simulink model "gm_test_prediction_without_delays"  (R2022a)
settings: Solver=FixedStepDiscrete  StartTime=0.0  StopTime=10.0  RelTol=1e-3
undefined symbols (not defined in the file or in its folder): f_c, L_d, L_q, L_x, L_y, p, psi_pm, R_ph
libraries: hdlmdlgenlib x2
(part 3 of 9)

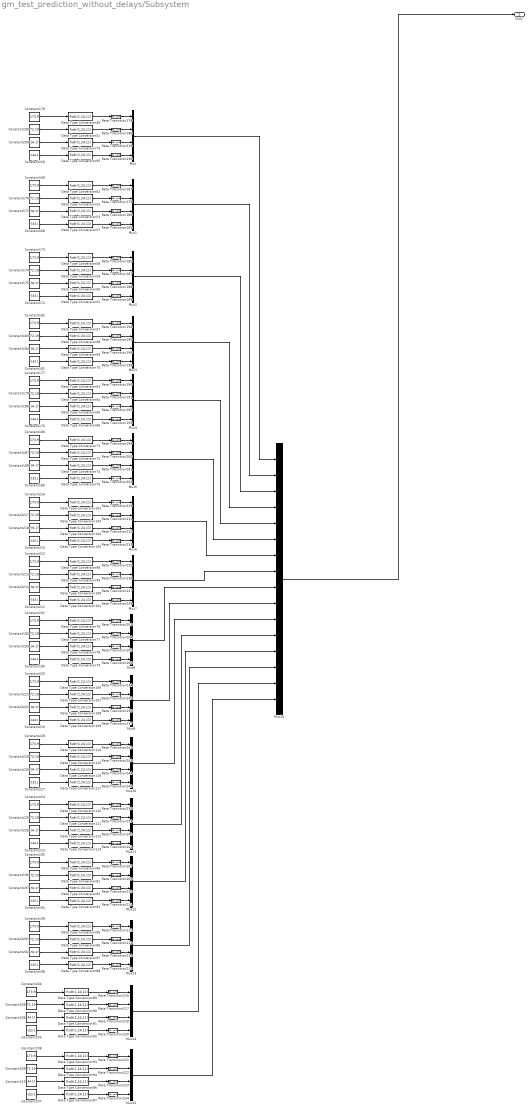
== system gm_test_prediction_without_delays/Subsystem ==
  Constant{156,168,172,176,181,185,190,194,198,203,207,211,215,219,223,227} (16 alike) : Constant  Value=-163.1
  Constant{169,173,177..178,182,186,191,195,199,204,208,212,216,220,224,228} (16 alike) : Constant  Value=173.9
  Constant{170,174,179,183,187,189,192,196,201,205,209,213,217,221,225,229} (16 alike) : Constant  Value=72.19
  Constant{171,175,180,184,188,193,197,200,202,206,210,214,218,222,226,230} (16 alike) : Constant  Value=-94.17
  Data Type Conversion{46,51..53,57..83,85..117} (64 alike) : DataTypeConversion  OutDataTypeStr=fixdt(1,24,11)  SaturateOnIntegerOverflow=off  RndMeth=Floor
  Mux{,1..15} (16 alike) : Mux
  Mux16 : Mux  Inputs=16
  Rate Transition{167,178..180,184..196,198..207,209..245} (64 alike) : RateTransition  OutPortSampleTime=Rt
  Out1 : Outport
  wires:
  Mux16/1 -> Out1/1
  Data Type Conversion65/1 -> Rate Transition192/1
  Data Type Conversion100/1 -> Rate Transition227/1
  Mux13/1 -> Mux16/14
  Constant204/1 -> Data Type Conversion89/1
  Rate Transition212/1 -> Mux13/1
  Constant220/1 -> Data Type Conversion106/1
  Constant202/1 -> Data Type Conversion87/1
  Constant218/1 -> Data Type Conversion104/1
  Rate Transition238/1 -> Mux11/1
  Constant224/1 -> Data Type Conversion110/1
  Rate Transition223/1 -> Mux15/3
  Constant177/1 -> Data Type Conversion63/1
  Constant183/1 -> Data Type Conversion68/1
  Data Type Conversion97/1 -> Rate Transition224/1
  Constant176/1 -> Data Type Conversion66/1
  Data Type Conversion74/1 -> Rate Transition201/1
  Data Type Conversion105/1 -> Rate Transition233/1
  Constant196/1 -> Data Type Conversion81/1
  Constant198/1 -> Data Type Conversion88/1
  Data Type Conversion115/1 -> Rate Transition243/1
  Constant225/1 -> Data Type Conversion111/1
  Constant222/1 -> Data Type Conversion108/1
  Data Type Conversion104/1 -> Rate Transition232/1
  Constant229/1 -> Data Type Conversion115/1
  Constant217/1 -> Data Type Conversion103/1
  Data Type Conversion72/1 -> Rate Transition200/1
  Data Type Conversion117/1 -> Rate Transition245/1
  Constant223/1 -> Data Type Conversion113/1
  Constant174/1 -> Data Type Conversion59/1
  Data Type Conversion110/1 -> Rate Transition238/1
  Data Type Conversion89/1 -> Rate Transition216/1
  Constant207/1 -> Data Type Conversion97/1
  Rate Transition185/1 -> Mux2/1
  Rate Transition196/1 -> Mux3/3
  Rate Transition230/1 -> Mux/4
  Data Type Conversion91/1 -> Rate Transition218/1
  Rate Transition167/1 -> Mux1/1
  Data Type Conversion85/1 -> Rate Transition212/1
  Rate Transition219/1 -> Mux/3
  Data Type Conversion102/1 -> Rate Transition229/1
  Constant156/1 -> Data Type Conversion95/1
  Constant228/1 -> Data Type Conversion114/1
  Rate Transition198/1 -> Mux3/4
  Rate Transition200/1 -> Mux5/2
  Data Type Conversion111/1 -> Rate Transition239/1
  Rate Transition192/1 -> Mux4/3
  Rate Transition190/1 -> Mux4/1
  Constant210/1 -> Data Type Conversion96/1
  Constant170/1 -> Data Type Conversion52/1
  Rate Transition195/1 -> Mux3/2
  Constant209/1 -> Data Type Conversion94/1
  Data Type Conversion93/1 -> Rate Transition221/1
  Data Type Conversion67/1 -> Rate Transition194/1
  Data Type Conversion73/1 -> Rate Transition219/1
  Constant184/1 -> Data Type Conversion69/1
  Rate Transition184/1 -> Mux1/4
  Data Type Conversion70/1 -> Rate Transition198/1
  Constant182/1 -> Data Type Conversion67/1
  Data Type Conversion75/1 -> Rate Transition202/1
  Constant189/1 -> Data Type Conversion51/1
  Constant206/1 -> Data Type Conversion91/1
  Constant192/1 -> Data Type Conversion77/1
  Data Type Conversion83/1 -> Rate Transition211/1
  Data Type Conversion59/1 -> Rate Transition187/1
  Mux14/1 -> Mux16/15
  Rate Transition241/1 -> Mux11/4
  Data Type Conversion107/1 -> Rate Transition235/1
  Rate Transition213/1 -> Mux13/2
  Constant172/1 -> Data Type Conversion61/1
  Constant221/1 -> Data Type Conversion107/1
  Data Type Conversion57/1 -> Rate Transition184/1
  Data Type Conversion61/1 -> Rate Transition189/1
  Constant197/1 -> Data Type Conversion82/1
  Rate Transition231/1 -> Mux6/2
  Constant173/1 -> Data Type Conversion58/1
  Constant190/1 -> Data Type Conversion79/1
  Constant230/1 -> Data Type Conversion116/1
  Constant193/1 -> Data Type Conversion78/1
  Rate Transition189/1 -> Mux2/4
  Rate Transition240/1 -> Mux11/3
  Rate Transition226/1 -> Mux7/2
  Data Type Conversion112/1 -> Rate Transition240/1
  Rate Transition239/1 -> Mux11/2
  Constant211/1 -> Data Type Conversion101/1
  Constant213/1 -> Data Type Conversion99/1
  Mux15/1 -> Mux16/16
  Data Type Conversion109/1 -> Rate Transition237/1
  Data Type Conversion46/1 -> Rate Transition178/1
  Data Type Conversion63/1 -> Rate Transition190/1
  Constant191/1 -> Data Type Conversion76/1
  Data Type Conversion80/1 -> Rate Transition207/1
  Constant168/1 -> Data Type Conversion57/1
  Constant195/1 -> Data Type Conversion80/1
  Constant194/1 -> Data Type Conversion83/1
  Data Type Conversion101/1 -> Rate Transition228/1
  Data Type Conversion77/1 -> Rate Transition204/1
  Data Type Conversion88/1 -> Rate Transition215/1
  Data Type Conversion96/1 -> Rate Transition223/1
  Rate Transition179/1 -> Mux1/2
  Data Type Conversion62/1 -> Rate Transition167/1
  Rate Transition234/1 -> Mux9/1
  Constant175/1 -> Data Type Conversion60/1
  Rate Transition225/1 -> Mux7/1
  Rate Transition218/1 -> Mux14/3
  Rate Transition220/1 -> Mux14/4
  Mux7/1 -> Mux16/8
  Rate Transition206/1 -> Mux8/4
  Data Type Conversion66/1 -> Rate Transition193/1
  Constant186/1 -> Data Type Conversion71/1
  Data Type Conversion98/1 -> Rate Transition225/1
  Rate Transition178/1 -> Mux/1
  Data Type Conversion81/1 -> Rate Transition209/1
  Data Type Conversion108/1 -> Rate Transition236/1
  Rate Transition237/1 -> Mux9/4
  Mux10/1 -> Mux16/11
  Constant205/1 -> Data Type Conversion90/1
  Mux4/1 -> Mux16/5
  Rate Transition245/1 -> Mux10/4
  Data Type Conversion52/1 -> Rate Transition179/1
  Rate Transition243/1 -> Mux10/2
  Constant208/1 -> Data Type Conversion93/1
  Constant185/1 -> Data Type Conversion75/1
  Constant216/1 -> Data Type Conversion102/1
  Data Type Conversion76/1 -> Rate Transition203/1
  Constant199/1 -> Data Type Conversion85/1
  Rate Transition209/1 -> Mux12/2
  Constant214/1 -> Data Type Conversion100/1
  Constant226/1 -> Data Type Conversion112/1
  Rate Transition228/1 -> Mux7/4
  Data Type Conversion69/1 -> Rate Transition196/1
  Constant201/1 -> Data Type Conversion86/1
  Constant171/1 -> Data Type Conversion53/1
  Rate Transition227/1 -> Mux7/3
  Rate Transition210/1 -> Mux12/3
  Rate Transition235/1 -> Mux9/2
  Rate Transition211/1 -> Mux12/4
  Mux8/1 -> Mux16/9
  Data Type Conversion79/1 -> Rate Transition206/1
  Mux1/1 -> Mux16/2
  Constant215/1 -> Data Type Conversion105/1
  Mux/1 -> Mux16/1
  Constant227/1 -> Data Type Conversion117/1
  Data Type Conversion68/1 -> Rate Transition195/1
  Constant178/1 -> Data Type Conversion46/1
  Mux6/1 -> Mux16/7
  Data Type Conversion53/1 -> Rate Transition180/1
  Data Type Conversion114/1 -> Rate Transition242/1
  Rate Transition232/1 -> Mux6/3
  Rate Transition224/1 -> Mux15/4
  Rate Transition186/1 -> Mux/2
  Rate Transition242/1 -> Mux10/1
  Rate Transition193/1 -> Mux4/4
  Rate Transition204/1 -> Mux8/2
  Constant212/1 -> Data Type Conversion98/1
  Constant181/1 -> Data Type Conversion70/1
  Rate Transition202/1 -> Mux5/4
  Rate Transition233/1 -> Mux6/4
  Data Type Conversion82/1 -> Rate Transition210/1
  Rate Transition188/1 -> Mux2/3
  Rate Transition216/1 -> Mux14/1
  Rate Transition244/1 -> Mux10/3
  Constant180/1 -> Data Type Conversion65/1
  Mux5/1 -> Mux16/6
  Constant219/1 -> Data Type Conversion109/1
  Data Type Conversion116/1 -> Rate Transition244/1
  Rate Transition203/1 -> Mux8/1
  Rate Transition215/1 -> Mux13/4
  Rate Transition205/1 -> Mux8/3
  Rate Transition194/1 -> Mux3/1
  Rate Transition229/1 -> Mux6/1
  Constant188/1 -> Data Type Conversion74/1
  Mux11/1 -> Mux16/12
  Mux9/1 -> Mux16/10
  Rate Transition221/1 -> Mux15/1
  Constant200/1 -> Data Type Conversion73/1
  Constant179/1 -> Data Type Conversion64/1
  Data Type Conversion94/1 -> Rate Transition222/1
  Mux2/1 -> Mux16/3
  Constant203/1 -> Data Type Conversion92/1
  Rate Transition217/1 -> Mux14/2
  Rate Transition191/1 -> Mux4/2
  Data Type Conversion99/1 -> Rate Transition226/1
  Constant187/1 -> Data Type Conversion72/1
  Data Type Conversion51/1 -> Rate Transition186/1
  Data Type Conversion71/1 -> Rate Transition199/1
  Data Type Conversion106/1 -> Rate Transition234/1
  Data Type Conversion86/1 -> Rate Transition213/1
  Data Type Conversion78/1 -> Rate Transition205/1
  Rate Transition199/1 -> Mux5/1
  Mux3/1 -> Mux16/4
  Rate Transition180/1 -> Mux1/3
  Rate Transition236/1 -> Mux9/3
  Rate Transition214/1 -> Mux13/3
  Data Type Conversion92/1 -> Rate Transition220/1
  Data Type Conversion64/1 -> Rate Transition191/1
  Data Type Conversion90/1 -> Rate Transition217/1
  Data Type Conversion87/1 -> Rate Transition214/1
  Data Type Conversion58/1 -> Rate Transition185/1
  Rate Transition187/1 -> Mux2/2
  Data Type Conversion60/1 -> Rate Transition188/1
  Rate Transition207/1 -> Mux12/1
  Data Type Conversion113/1 -> Rate Transition241/1
  Mux12/1 -> Mux16/13
  Data Type Conversion103/1 -> Rate Transition231/1
  Rate Transition201/1 -> Mux5/3
  Rate Transition222/1 -> Mux15/2
  Data Type Conversion95/1 -> Rate Transition230/1
  Constant169/1 -> Data Type Conversion62/1

== system gm_test_prediction_without_delays/Prediction_and_cost_function1/Compare To Constant ==
  u : Inport  OutDataTypeStr=fixdt(1,32,0,'DataTypeOverride', 'Off')  SampleTime=1e-08
  Compare : RelationalOperator  Operator=<=  OutDataTypeStr=boolean
  Constant : Constant  DisableCoverage=on  Value=const  OutDataTypeStr=Inherit: Inherit via back propagation  SampleTime=-1
  y : Outport  SampleTime=1e-08
  wires:
  Compare/1 -> y/1
  Constant/1 -> Compare/2
  u/1 -> Compare/1

== system gm_test_prediction_without_delays/Prediction_and_cost_function1/Data Type Conversion1 ==
  In1 : Inport
  Data Type Conversion1 : DataTypeConversion  OutDataTypeStr=single  RndMeth=Nearest  SampleTime=1e-08  SaturateOnIntegerOverflow=off
  Data Type Conversion1_pd1 : Delay  DelayLength=6
  Out1 : Outport
  wires:
  In1/1 -> Data Type Conversion1/1
  Data Type Conversion1/1 -> Data Type Conversion1_pd1/1
  Data Type Conversion1_pd1/1 -> Out1/1

== system gm_test_prediction_without_delays/Prediction_and_cost_function1/Data Type Conversion10 ==
  In1 : Inport
  Data Type Conversion10 : DataTypeConversion  OutDataTypeStr=single  RndMeth=Nearest  SampleTime=1e-08  SaturateOnIntegerOverflow=off
  Data Type Conversion10_pd1 : Delay  DelayLength=6
  Out1 : Outport
  wires:
  In1/1 -> Data Type Conversion10/1
  Data Type Conversion10/1 -> Data Type Conversion10_pd1/1
  Data Type Conversion10_pd1/1 -> Out1/1

== system gm_test_prediction_without_delays/Prediction_and_cost_function1/Data Type Conversion18 ==
  In1 : Inport
  Data Type Conversion18 : DataTypeConversion  OutDataTypeStr=fixdt(1, 18, 11)  RndMeth=Nearest  SampleTime=1e-08  SaturateOnIntegerOverflow=off
  Data Type Conversion18_pd1 : Delay  DelayLength=6
  Out1 : Outport
  wires:
  In1/1 -> Data Type Conversion18/1
  Data Type Conversion18/1 -> Data Type Conversion18_pd1/1
  Data Type Conversion18_pd1/1 -> Out1/1

== system gm_test_prediction_without_delays/Prediction_and_cost_function1/Data Type Conversion4 ==
  In1 : Inport
  Data Type Conversion4 : DataTypeConversion  OutDataTypeStr=single  RndMeth=Nearest  SampleTime=1e-08  SaturateOnIntegerOverflow=off
  Data Type Conversion4_pd1 : Delay  DelayLength=6
  Out1 : Outport
  wires:
  In1/1 -> Data Type Conversion4/1
  Data Type Conversion4/1 -> Data Type Conversion4_pd1/1
  Data Type Conversion4_pd1/1 -> Out1/1

== system gm_test_prediction_without_delays/Prediction_and_cost_function1/Data Type Conversion7 ==
  In1 : Inport
  Data Type Conversion7 : DataTypeConversion  OutDataTypeStr=single  RndMeth=Nearest  SampleTime=1e-08  SaturateOnIntegerOverflow=off
  Data Type Conversion7_pd1 : Delay  DelayLength=6
  Out1 : Outport
  wires:
  In1/1 -> Data Type Conversion7/1
  Data Type Conversion7/1 -> Data Type Conversion7_pd1/1
  Data Type Conversion7_pd1/1 -> Out1/1

== system gm_test_prediction_without_delays/Prediction_and_cost_function1/Data Type Conversion8 ==
  In1 : Inport
  Data Type Conversion8 : DataTypeConversion  OutDataTypeStr=single  RndMeth=Nearest  SampleTime=1e-08  SaturateOnIntegerOverflow=off
  Data Type Conversion8_pd1 : Delay  DelayLength=6
  Out1 : Outport
  wires:
  In1/1 -> Data Type Conversion8/1
  Data Type Conversion8/1 -> Data Type Conversion8_pd1/1
  Data Type Conversion8_pd1/1 -> Out1/1

== system gm_test_prediction_without_delays/Prediction_and_cost_function1/Data Type Conversion9 ==
  In1 : Inport
  Data Type Conversion9 : DataTypeConversion  OutDataTypeStr=single  RndMeth=Nearest  SampleTime=1e-08  SaturateOnIntegerOverflow=off
  Data Type Conversion9_pd1 : Delay  DelayLength=6
  Out1 : Outport
  wires:
  In1/1 -> Data Type Conversion9/1
  Data Type Conversion9/1 -> Data Type Conversion9_pd1/1
  Data Type Conversion9_pd1/1 -> Out1/1

== system gm_test_prediction_without_delays/Prediction_and_cost_function1/Detect Rise Positive ==
  note: Edge
  note: U(k)
  U : Inport  OutDataTypeStr=boolean  SampleTime=1e-08
  Delay Input1 : UnitDelay  Description=Store in Global RAM  DisableCoverage=on  InitialCondition=vinit  SampleTime=-1  HasFrameUpgradeWarning=on
  FixPt Relational Operator : RelationalOperator  Operator=>  OutDataTypeStr=boolean  ZeroCross=off  InputSameDT=off
  Positive : Subsystem  mask(Compare To Zero){relop=>, OutDataTypeStr=boolean, ZeroCross=off}
      mask prompts: relop "Simulink:masks:Operator_MP"; OutDataTypeStr "Simulink:masks:OutputDataType_MP"; ZeroCross "Simulink:masks:EnableZerocrossingDetection_MP"
      mask help: Simulink:masks:CompareToZero_MD
      mask init:
      | OutDataTypeStr = 'boolean';
      | ZeroCross = 'off';
      | blkName = 'test_prediction_without_delays/Prediction_and_cost_function1/Detect Rise\nPositive/Positive';
      | relop = '>';
      | setValue = 'boolean';
      mask TypeOptions relop: == | ~= | < | <= | >= | >
      mask TypeOptions OutDataTypeStr: Simulink:masks:uint8 | Simulink:masks:boolean
      mask Callback ZeroCross: sl('zeroCrossEnable', gcbh);
      mask Display: disp([relop,' 0'])
  Y : Outport  SampleTime=1e-08
  wires:
  Delay Input1/1 -> FixPt Relational Operator/2
  FixPt Relational Operator/1 -> Y/1
  Positive/1(y) -> FixPt Relational Operator/1, Delay Input1/1
  U/1 -> Positive/1(u)

== system gm_test_prediction_without_delays/Prediction_and_cost_function1/Detect Rise Positive1 ==
  note: Edge
  note: U(k)
  U : Inport  OutDataTypeStr=boolean  SampleTime=1e-08
  Delay Input1 : UnitDelay  Description=Store in Global RAM  DisableCoverage=on  InitialCondition=vinit  SampleTime=-1  HasFrameUpgradeWarning=on
  FixPt Relational Operator : RelationalOperator  Operator=>  OutDataTypeStr=boolean  ZeroCross=off  InputSameDT=off
  Positive : Subsystem  mask(Compare To Zero){relop=>, OutDataTypeStr=boolean, ZeroCross=off}
      mask prompts: relop "Simulink:masks:Operator_MP"; OutDataTypeStr "Simulink:masks:OutputDataType_MP"; ZeroCross "Simulink:masks:EnableZerocrossingDetection_MP"
      mask help: Simulink:masks:CompareToZero_MD
      mask init:
      | OutDataTypeStr = 'boolean';
      | ZeroCross = 'off';
      | blkName = 'test_prediction_without_delays/Prediction_and_cost_function1/Detect Rise\nPositive1/Positive';
      | relop = '>';
      | setValue = 'boolean';
      mask TypeOptions relop: == | ~= | < | <= | >= | >
      mask TypeOptions OutDataTypeStr: Simulink:masks:uint8 | Simulink:masks:boolean
      mask Callback ZeroCross: sl('zeroCrossEnable', gcbh);
      mask Display: disp([relop,' 0'])
  Y : Outport  SampleTime=1e-08
  wires:
  Delay Input1/1 -> FixPt Relational Operator/2
  FixPt Relational Operator/1 -> Y/1
  Positive/1(y) -> FixPt Relational Operator/1, Delay Input1/1
  U/1 -> Positive/1(u)

== system gm_test_prediction_without_delays/Prediction_and_cost_function1/Detect Rise Positive2 ==
  note: Edge
  note: U(k)
  U : Inport  OutDataTypeStr=boolean  SampleTime=1e-08
  Delay Input1 : UnitDelay  Description=Store in Global RAM  DisableCoverage=on  InitialCondition=vinit  SampleTime=-1  HasFrameUpgradeWarning=on
  FixPt Relational Operator : RelationalOperator  Operator=>  OutDataTypeStr=boolean  ZeroCross=off  InputSameDT=off
  Positive : Subsystem  mask(Compare To Zero){relop=>, OutDataTypeStr=boolean, ZeroCross=off}
      mask prompts: relop "Simulink:masks:Operator_MP"; OutDataTypeStr "Simulink:masks:OutputDataType_MP"; ZeroCross "Simulink:masks:EnableZerocrossingDetection_MP"
      mask help: Simulink:masks:CompareToZero_MD
      mask init:
      | OutDataTypeStr = 'boolean';
      | ZeroCross = 'off';
      | blkName = 'test_prediction_without_delays/Prediction_and_cost_function1/Detect Rise\nPositive2/Positive';
      | relop = '>';
      | setValue = 'boolean';
      mask TypeOptions relop: == | ~= | < | <= | >= | >
      mask TypeOptions OutDataTypeStr: Simulink:masks:uint8 | Simulink:masks:boolean
      mask Callback ZeroCross: sl('zeroCrossEnable', gcbh);
      mask Display: disp([relop,' 0'])
  Y : Outport  SampleTime=1e-08
  wires:
  Delay Input1/1 -> FixPt Relational Operator/2
  FixPt Relational Operator/1 -> Y/1
  Positive/1(y) -> FixPt Relational Operator/1, Delay Input1/1
  U/1 -> Positive/1(u)

== system gm_test_prediction_without_delays/Prediction_and_cost_function1/Product ==
  In1 : Inport
  In2 : Inport  Port=2
  Product : Product  Inputs=**  OutDataTypeStr=single  SampleTime=1e-08
  Product_pd1 : Delay  DelayLength=6
  Out1 : Outport
  wires:
  In1/1 -> Product/1
  In2/1 -> Product/2
  Product/1 -> Product_pd1/1
  Product_pd1/1 -> Out1/1

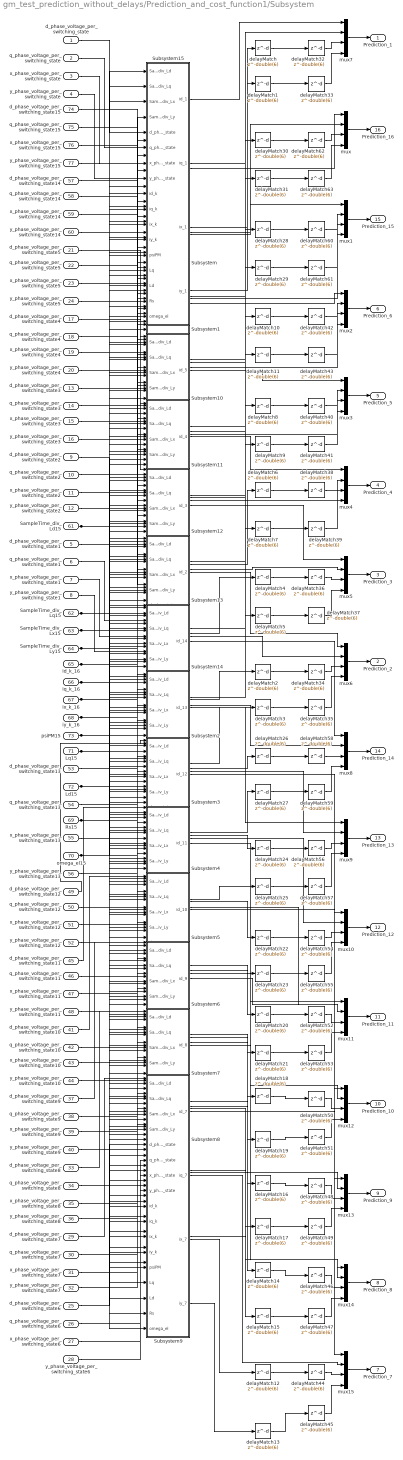
== system gm_test_prediction_without_delays/Prediction_and_cost_function1/Subsystem ==
  d_phase_voltage_per_switching_state : Inport  OutDataTypeStr=single  PortDimensions=1  SampleTime=1e-08
  q_phase_voltage_per_switching_state : Inport  Port=2  OutDataTypeStr=single  PortDimensions=1  SampleTime=1e-08
  x_phase_voltage_per_switching_state : Inport  Port=3  OutDataTypeStr=single  PortDimensions=1  SampleTime=1e-08
  y_phase_voltage_per_switching_state : Inport  Port=4  OutDataTypeStr=single  PortDimensions=1  SampleTime=1e-08
  d_phase_voltage_per_switching_state1 : Inport  Port=5  OutDataTypeStr=single  PortDimensions=1  SampleTime=1e-08
  q_phase_voltage_per_switching_state1 : Inport  Port=6  OutDataTypeStr=single  PortDimensions=1  SampleTime=1e-08
  x_phase_voltage_per_switching_state1 : Inport  Port=7  OutDataTypeStr=single  PortDimensions=1  SampleTime=1e-08
  y_phase_voltage_per_switching_state1 : Inport  Port=8  OutDataTypeStr=single  PortDimensions=1  SampleTime=1e-08
  d_phase_voltage_per_switching_state2 : Inport  Port=9  OutDataTypeStr=single  PortDimensions=1  SampleTime=1e-08
  q_phase_voltage_per_switching_state2 : Inport  Port=10  OutDataTypeStr=single  PortDimensions=1  SampleTime=1e-08
  x_phase_voltage_per_switching_state2 : Inport  Port=11  OutDataTypeStr=single  PortDimensions=1  SampleTime=1e-08
  y_phase_voltage_per_switching_state2 : Inport  Port=12  OutDataTypeStr=single  PortDimensions=1  SampleTime=1e-08
  d_phase_voltage_per_switching_state3 : Inport  Port=13  OutDataTypeStr=single  PortDimensions=1  SampleTime=1e-08
  q_phase_voltage_per_switching_state3 : Inport  Port=14  OutDataTypeStr=single  PortDimensions=1  SampleTime=1e-08
  x_phase_voltage_per_switching_state3 : Inport  Port=15  OutDataTypeStr=single  PortDimensions=1  SampleTime=1e-08
  y_phase_voltage_per_switching_state3 : Inport  Port=16  OutDataTypeStr=single  PortDimensions=1  SampleTime=1e-08
  d_phase_voltage_per_switching_state4 : Inport  Port=17  OutDataTypeStr=single  PortDimensions=1  SampleTime=1e-08
  q_phase_voltage_per_switching_state4 : Inport  Port=18  OutDataTypeStr=single  PortDimensions=1  SampleTime=1e-08
  x_phase_voltage_per_switching_state4 : Inport  Port=19  OutDataTypeStr=single  PortDimensions=1  SampleTime=1e-08
  y_phase_voltage_per_switching_state4 : Inport  Port=20  OutDataTypeStr=single  PortDimensions=1  SampleTime=1e-08
  d_phase_voltage_per_switching_state5 : Inport  Port=21  OutDataTypeStr=single  PortDimensions=1  SampleTime=1e-08
  q_phase_voltage_per_switching_state5 : Inport  Port=22  OutDataTypeStr=single  PortDimensions=1  SampleTime=1e-08
  x_phase_voltage_per_switching_state5 : Inport  Port=23  OutDataTypeStr=single  PortDimensions=1  SampleTime=1e-08
  y_phase_voltage_per_switching_state5 : Inport  Port=24  OutDataTypeStr=single  PortDimensions=1  SampleTime=1e-08
  d_phase_voltage_per_switching_state6 : Inport  Port=25  OutDataTypeStr=single  PortDimensions=1  SampleTime=1e-08
  q_phase_voltage_per_switching_state6 : Inport  Port=26  OutDataTypeStr=single  PortDimensions=1  SampleTime=1e-08
  x_phase_voltage_per_switching_state6 : Inport  Port=27  OutDataTypeStr=single  PortDimensions=1  SampleTime=1e-08
  y_phase_voltage_per_switching_state6 : Inport  Port=28  OutDataTypeStr=single  PortDimensions=1  SampleTime=1e-08
  d_phase_voltage_per_switching_state7 : Inport  Port=29  OutDataTypeStr=single  PortDimensions=1  SampleTime=1e-08
  q_phase_voltage_per_switching_state7 : Inport  Port=30  OutDataTypeStr=single  PortDimensions=1  SampleTime=1e-08
  x_phase_voltage_per_switching_state7 : Inport  Port=31  OutDataTypeStr=single  PortDimensions=1  SampleTime=1e-08
  y_phase_voltage_per_switching_state7 : Inport  Port=32  OutDataTypeStr=single  PortDimensions=1  SampleTime=1e-08
  d_phase_voltage_per_switching_state8 : Inport  Port=33  OutDataTypeStr=single  PortDimensions=1  SampleTime=1e-08
  q_phase_voltage_per_switching_state8 : Inport  Port=34  OutDataTypeStr=single  PortDimensions=1  SampleTime=1e-08
  x_phase_voltage_per_switching_state8 : Inport  Port=35  OutDataTypeStr=single  PortDimensions=1  SampleTime=1e-08
  y_phase_voltage_per_switching_state8 : Inport  Port=36  OutDataTypeStr=single  PortDimensions=1  SampleTime=1e-08
  d_phase_voltage_per_switching_state9 : Inport  Port=37  OutDataTypeStr=single  PortDimensions=1  SampleTime=1e-08
  q_phase_voltage_per_switching_state9 : Inport  Port=38  OutDataTypeStr=single  PortDimensions=1  SampleTime=1e-08
  x_phase_voltage_per_switching_state9 : Inport  Port=39  OutDataTypeStr=single  PortDimensions=1  SampleTime=1e-08
  y_phase_voltage_per_switching_state9 : Inport  Port=40  OutDataTypeStr=single  PortDimensions=1  SampleTime=1e-08
  d_phase_voltage_per_switching_state10 : Inport  Port=41  OutDataTypeStr=single  PortDimensions=1  SampleTime=1e-08
  q_phase_voltage_per_switching_state10 : Inport  Port=42  OutDataTypeStr=single  PortDimensions=1  SampleTime=1e-08
  x_phase_voltage_per_switching_state10 : Inport  Port=43  OutDataTypeStr=single  PortDimensions=1  SampleTime=1e-08
  y_phase_voltage_per_switching_state10 : Inport  Port=44  OutDataTypeStr=single  PortDimensions=1  SampleTime=1e-08
  d_phase_voltage_per_switching_state11 : Inport  Port=45  OutDataTypeStr=single  PortDimensions=1  SampleTime=1e-08
  q_phase_voltage_per_switching_state11 : Inport  Port=46  OutDataTypeStr=single  PortDimensions=1  SampleTime=1e-08
  x_phase_voltage_per_switching_state11 : Inport  Port=47  OutDataTypeStr=single  PortDimensions=1  SampleTime=1e-08
  y_phase_voltage_per_switching_state11 : Inport  Port=48  OutDataTypeStr=single  PortDimensions=1  SampleTime=1e-08
  d_phase_voltage_per_switching_state12 : Inport  Port=49  OutDataTypeStr=single  PortDimensions=1  SampleTime=1e-08
  q_phase_voltage_per_switching_state12 : Inport  Port=50  OutDataTypeStr=single  PortDimensions=1  SampleTime=1e-08
  x_phase_voltage_per_switching_state12 : Inport  Port=51  OutDataTypeStr=single  PortDimensions=1  SampleTime=1e-08
  y_phase_voltage_per_switching_state12 : Inport  Port=52  OutDataTypeStr=single  PortDimensions=1  SampleTime=1e-08
  d_phase_voltage_per_switching_state13 : Inport  Port=53  OutDataTypeStr=single  PortDimensions=1  SampleTime=1e-08
  q_phase_voltage_per_switching_state13 : Inport  Port=54  OutDataTypeStr=single  PortDimensions=1  SampleTime=1e-08
  x_phase_voltage_per_switching_state13 : Inport  Port=55  OutDataTypeStr=single  PortDimensions=1  SampleTime=1e-08
  y_phase_voltage_per_switching_state13 : Inport  Port=56  OutDataTypeStr=single  PortDimensions=1  SampleTime=1e-08
  d_phase_voltage_per_switching_state14 : Inport  Port=57  OutDataTypeStr=single  PortDimensions=1  SampleTime=1e-08
  q_phase_voltage_per_switching_state14 : Inport  Port=58  OutDataTypeStr=single  PortDimensions=1  SampleTime=1e-08
  x_phase_voltage_per_switching_state14 : Inport  Port=59  OutDataTypeStr=single  PortDimensions=1  SampleTime=1e-08
  y_phase_voltage_per_switching_state14 : Inport  Port=60  OutDataTypeStr=single  PortDimensions=1  SampleTime=1e-08
  SampleTime_div_Ld15 : Inport  Port=61  OutDataTypeStr=single  PortDimensions=1  SampleTime=1e-08
  SampleTime_div_Lq15 : Inport  Port=62  OutDataTypeStr=single  PortDimensions=1  SampleTime=1e-08
  SampleTime_div_Lx15 : Inport  Port=63  OutDataTypeStr=single  PortDimensions=1  SampleTime=1e-08
  SampleTime_div_Ly15 : Inport  Port=64  OutDataTypeStr=single  PortDimensions=1  SampleTime=1e-08
  id_k_16 : Inport  Port=65  OutDataTypeStr=single  PortDimensions=1  SampleTime=1e-08
  iq_k_16 : Inport  Port=66  OutDataTypeStr=single  PortDimensions=1  SampleTime=1e-08
  ix_k_16 : Inport  Port=67  OutDataTypeStr=single  PortDimensions=1  SampleTime=1e-08
  iy_k_16 : Inport  Port=68  OutDataTypeStr=single  PortDimensions=1  SampleTime=1e-08
  Rs15 : Inport  Port=69  OutDataTypeStr=single  PortDimensions=1  SampleTime=1e-08
  omega_el15 : Inport  Port=70  OutDataTypeStr=single  PortDimensions=1  SampleTime=1e-08
  Lq15 : Inport  Port=71  OutDataTypeStr=single  PortDimensions=1  SampleTime=1e-08
  Ld15 : Inport  Port=72  OutDataTypeStr=single  PortDimensions=1  SampleTime=1e-08
  psiPM15 : Inport  Port=73  OutDataTypeStr=single  PortDimensions=1  SampleTime=1e-08
  d_phase_voltage_per_switching_state15 : Inport  Port=74  OutDataTypeStr=single  PortDimensions=1  SampleTime=1e-08
  q_phase_voltage_per_switching_state15 : Inport  Port=75  OutDataTypeStr=single  PortDimensions=1  SampleTime=1e-08
  x_phase_voltage_per_switching_state15 : Inport  Port=76  OutDataTypeStr=single  PortDimensions=1  SampleTime=1e-08
  y_phase_voltage_per_switching_state15 : Inport  Port=77  OutDataTypeStr=single  PortDimensions=1  SampleTime=1e-08
  Subsystem : Subsystem
  Subsystem1 : Subsystem
  Subsystem10 : Subsystem
  Subsystem11 : Subsystem
  Subsystem12 : Subsystem
  Subsystem13 : Subsystem
  Subsystem14 : Subsystem
  Subsystem15 : Subsystem
  Subsystem2 : Subsystem
  Subsystem3 : Subsystem
  Subsystem4 : Subsystem
  Subsystem5 : Subsystem
  Subsystem6 : Subsystem
  Subsystem7 : Subsystem
  Subsystem8 : Subsystem
  Subsystem9 : Subsystem
  delayMatch{,1..63} (64 alike) : Delay  DelayLength=double(6)  InitialCondition=0  SampleTime=1e-08
  mux{,1..15} (16 alike) : Mux
  Prediction_1 : Outport  SampleTime=1e-08
  Prediction_2 : Outport  Port=2  SampleTime=1e-08
  Prediction_3 : Outport  Port=3  SampleTime=1e-08
  Prediction_4 : Outport  Port=4  SampleTime=1e-08
  Prediction_5 : Outport  Port=5  SampleTime=1e-08
  Prediction_6 : Outport  Port=6  SampleTime=1e-08
  Prediction_7 : Outport  Port=7  SampleTime=1e-08
  Prediction_8 : Outport  Port=8  SampleTime=1e-08
  Prediction_9 : Outport  Port=9  SampleTime=1e-08
  Prediction_10 : Outport  Port=10  SampleTime=1e-08
  Prediction_11 : Outport  Port=11  SampleTime=1e-08
  Prediction_12 : Outport  Port=12  SampleTime=1e-08
  Prediction_13 : Outport  Port=13  SampleTime=1e-08
  Prediction_14 : Outport  Port=14  SampleTime=1e-08
  Prediction_15 : Outport  Port=15  SampleTime=1e-08
  Prediction_16 : Outport  Port=16  SampleTime=1e-08
  wires:
  mux/1 -> Prediction_16/1
  mux1/1 -> Prediction_15/1
  mux2/1 -> Prediction_6/1
  mux3/1 -> Prediction_5/1
  mux4/1 -> Prediction_4/1
  mux5/1 -> Prediction_3/1
  mux6/1 -> Prediction_2/1
  mux7/1 -> Prediction_1/1
  mux8/1 -> Prediction_14/1
  mux9/1 -> Prediction_13/1
  mux10/1 -> Prediction_12/1
  mux11/1 -> Prediction_11/1
  mux12/1 -> Prediction_10/1
  mux13/1 -> Prediction_9/1
  mux14/1 -> Prediction_8/1
  mux15/1 -> Prediction_7/1
  Subsystem/2(iq_16) -> mux/2
  delayMatch62/1 -> mux/3
  delayMatch63/1 -> mux/4
  Subsystem1/2(iq_15) -> mux1/2
  delayMatch60/1 -> mux1/3
  delayMatch61/1 -> mux1/4
  Subsystem10/2(iq_6) -> mux2/2
  delayMatch42/1 -> mux2/3
  delayMatch43/1 -> mux2/4
  Subsystem11/2(iq_5) -> mux3/2
  delayMatch40/1 -> mux3/3
  delayMatch41/1 -> mux3/4
  Subsystem12/2(iq_4) -> mux4/2
  delayMatch38/1 -> mux4/3
  delayMatch39/1 -> mux4/4
  Subsystem13/2(iq_3) -> mux5/2
  delayMatch36/1 -> mux5/3
  delayMatch37/1 -> mux5/4
  Subsystem14/2(iq_2) -> mux6/2
  delayMatch34/1 -> mux6/3
  delayMatch35/1 -> mux6/4
  Subsystem15/2(iq_1) -> mux7/2
  delayMatch32/1 -> mux7/3
  delayMatch33/1 -> mux7/4
  Subsystem2/2(iq_14) -> mux8/2
  delayMatch58/1 -> mux8/3
  delayMatch59/1 -> mux8/4
  Subsystem3/2(iq_13) -> mux9/2
  delayMatch56/1 -> mux9/3
  delayMatch57/1 -> mux9/4
  Subsystem4/2(iq_12) -> mux10/2
  delayMatch54/1 -> mux10/3
  delayMatch55/1 -> mux10/4
  Subsystem5/2(iq_11) -> mux11/2
  delayMatch52/1 -> mux11/3
  delayMatch53/1 -> mux11/4
  Subsystem6/2(iq_10) -> mux12/2
  delayMatch50/1 -> mux12/3
  delayMatch51/1 -> mux12/4
  Subsystem7/2(iq_9) -> mux13/2
  delayMatch48/1 -> mux13/3
  delayMatch49/1 -> mux13/4
  Subsystem8/2(iq_8) -> mux14/2
  delayMatch46/1 -> mux14/3
  delayMatch47/1 -> mux14/4
  Subsystem9/2(iq_7) -> mux15/2
  delayMatch44/1 -> mux15/3
  delayMatch45/1 -> mux15/4
  Subsystem15/1(id_1) -> mux7/1
  Subsystem15/3(ix_1) -> delayMatch/1
  Subsystem15/4(iy_1) -> delayMatch1/1
  Subsystem14/1(id_2) -> mux6/1
  Subsystem14/3(ix_2) -> delayMatch2/1
  Subsystem14/4(iy_2) -> delayMatch3/1
  Subsystem13/1(id_3) -> mux5/1
  Subsystem13/3(ix_3) -> delayMatch4/1
  Subsystem13/4(iy_3) -> delayMatch5/1
  Subsystem12/1(id_4) -> mux4/1
  Subsystem12/3(ix_4) -> delayMatch6/1
  Subsystem12/4(iy_4) -> delayMatch7/1
  Subsystem11/1(id_5) -> mux3/1
  Subsystem11/3(ix_5) -> delayMatch8/1
  Subsystem11/4(iy_5) -> delayMatch9/1
  Subsystem10/1(id_6) -> mux2/1
  Subsystem10/3(ix_6) -> delayMatch10/1
  Subsystem10/4(iy_6) -> delayMatch11/1
  Subsystem9/1(id_7) -> mux15/1
  Subsystem9/3(ix_7) -> delayMatch12/1
  Subsystem9/4(iy_7) -> delayMatch13/1
  Subsystem8/1(id_8) -> mux14/1
  Subsystem8/3(ix_8) -> delayMatch14/1
  Subsystem8/4(iy_8) -> delayMatch15/1
  Subsystem7/1(id_9) -> mux13/1
  Subsystem7/3(ix_9) -> delayMatch16/1
  Subsystem7/4(iy_9) -> delayMatch17/1
  Subsystem6/1(id_10) -> mux12/1
  Subsystem6/3(ix_10) -> delayMatch18/1
  Subsystem6/4(iy_10) -> delayMatch19/1
  Subsystem5/1(id_11) -> mux11/1
  Subsystem5/3(ix_11) -> delayMatch20/1
  Subsystem5/4(iy_11) -> delayMatch21/1
  Subsystem4/1(id_12) -> mux10/1
  Subsystem4/3(ix_12) -> delayMatch22/1
  Subsystem4/4(iy_12) -> delayMatch23/1
  Subsystem3/1(id_13) -> mux9/1
  Subsystem3/3(ix_13) -> delayMatch24/1
  Subsystem3/4(iy_13) -> delayMatch25/1
  Subsystem2/1(id_14) -> mux8/1
  Subsystem2/3(ix_14) -> delayMatch26/1
  Subsystem2/4(iy_14) -> delayMatch27/1
  Subsystem1/1(id_15) -> mux1/1
  Subsystem1/3(ix_15) -> delayMatch28/1
  Subsystem1/4(iy_15) -> delayMatch29/1
  Subsystem/1(id_16) -> mux/1
  Subsystem/3(ix_16) -> delayMatch30/1
  Subsystem/4(iy_16) -> delayMatch31/1
  delayMatch/1 -> delayMatch32/1
  delayMatch1/1 -> delayMatch33/1
  delayMatch2/1 -> delayMatch34/1
  delayMatch3/1 -> delayMatch35/1
  delayMatch4/1 -> delayMatch36/1
  delayMatch5/1 -> delayMatch37/1
  delayMatch6/1 -> delayMatch38/1
  delayMatch7/1 -> delayMatch39/1
  delayMatch8/1 -> delayMatch40/1
  delayMatch9/1 -> delayMatch41/1
  delayMatch10/1 -> delayMatch42/1
  delayMatch11/1 -> delayMatch43/1
  delayMatch12/1 -> delayMatch44/1
  delayMatch13/1 -> delayMatch45/1
  delayMatch14/1 -> delayMatch46/1
  delayMatch15/1 -> delayMatch47/1
  delayMatch16/1 -> delayMatch48/1
  delayMatch17/1 -> delayMatch49/1
  delayMatch18/1 -> delayMatch50/1
  delayMatch19/1 -> delayMatch51/1
  delayMatch20/1 -> delayMatch52/1
  delayMatch21/1 -> delayMatch53/1
  delayMatch22/1 -> delayMatch54/1
  delayMatch23/1 -> delayMatch55/1
  delayMatch24/1 -> delayMatch56/1
  delayMatch25/1 -> delayMatch57/1
  delayMatch26/1 -> delayMatch58/1
  delayMatch27/1 -> delayMatch59/1
  delayMatch28/1 -> delayMatch60/1
  delayMatch29/1 -> delayMatch61/1
  delayMatch30/1 -> delayMatch62/1
  delayMatch31/1 -> delayMatch63/1
  d_phase_voltage_per_switching_state/1 -> Subsystem15/5(d_phase_voltage_per_switching_state)
  q_phase_voltage_per_switching_state/1 -> Subsystem15/6(q_phase_voltage_per_switching_state)
  x_phase_voltage_per_switching_state/1 -> Subsystem15/7(x_phase_voltage_per_switching_state)
  y_phase_voltage_per_switching_state/1 -> Subsystem15/8(y_phase_voltage_per_switching_state)
  d_phase_voltage_per_switching_state1/1 -> Subsystem14/5(d_phase_voltage_per_switching_state)
  q_phase_voltage_per_switching_state1/1 -> Subsystem14/6(q_phase_voltage_per_switching_state)
  x_phase_voltage_per_switching_state1/1 -> Subsystem14/7(x_phase_voltage_per_switching_state)
  y_phase_voltage_per_switching_state1/1 -> Subsystem14/8(y_phase_voltage_per_switching_state)
  d_phase_voltage_per_switching_state2/1 -> Subsystem13/5(d_phase_voltage_per_switching_state)
  q_phase_voltage_per_switching_state2/1 -> Subsystem13/6(q_phase_voltage_per_switching_state)
  x_phase_voltage_per_switching_state2/1 -> Subsystem13/7(x_phase_voltage_per_switching_state)
  y_phase_voltage_per_switching_state2/1 -> Subsystem13/8(y_phase_voltage_per_switching_state)
  d_phase_voltage_per_switching_state3/1 -> Subsystem12/5(d_phase_voltage_per_switching_state)
  q_phase_voltage_per_switching_state3/1 -> Subsystem12/6(q_phase_voltage_per_switching_state)
  x_phase_voltage_per_switching_state3/1 -> Subsystem12/7(x_phase_voltage_per_switching_state)
  y_phase_voltage_per_switching_state3/1 -> Subsystem12/8(y_phase_voltage_per_switching_state)
  d_phase_voltage_per_switching_state4/1 -> Subsystem11/5(d_phase_voltage_per_switching_state)
  q_phase_voltage_per_switching_state4/1 -> Subsystem11/6(q_phase_voltage_per_switching_state)
  x_phase_voltage_per_switching_state4/1 -> Subsystem11/7(x_phase_voltage_per_switching_state)
  y_phase_voltage_per_switching_state4/1 -> Subsystem11/8(y_phase_voltage_per_switching_state)
  d_phase_voltage_per_switching_state5/1 -> Subsystem10/5(d_phase_voltage_per_switching_state)
  q_phase_voltage_per_switching_state5/1 -> Subsystem10/6(q_phase_voltage_per_switching_state)
  x_phase_voltage_per_switching_state5/1 -> Subsystem10/7(x_phase_voltage_per_switching_state)
  y_phase_voltage_per_switching_state5/1 -> Subsystem10/8(y_phase_voltage_per_switching_state)
  d_phase_voltage_per_switching_state6/1 -> Subsystem9/5(d_phase_voltage_per_switching_state)
  q_phase_voltage_per_switching_state6/1 -> Subsystem9/6(q_phase_voltage_per_switching_state)
  x_phase_voltage_per_switching_state6/1 -> Subsystem9/7(x_phase_voltage_per_switching_state)
  y_phase_voltage_per_switching_state6/1 -> Subsystem9/8(y_phase_voltage_per_switching_state)
  d_phase_voltage_per_switching_state7/1 -> Subsystem8/5(d_phase_voltage_per_switching_state)
  q_phase_voltage_per_switching_state7/1 -> Subsystem8/6(q_phase_voltage_per_switching_state)
  x_phase_voltage_per_switching_state7/1 -> Subsystem8/7(x_phase_voltage_per_switching_state)
  y_phase_voltage_per_switching_state7/1 -> Subsystem8/8(y_phase_voltage_per_switching_state)
  d_phase_voltage_per_switching_state8/1 -> Subsystem7/5(d_phase_voltage_per_switching_state)
  q_phase_voltage_per_switching_state8/1 -> Subsystem7/6(q_phase_voltage_per_switching_state)
  x_phase_voltage_per_switching_state8/1 -> Subsystem7/7(x_phase_voltage_per_switching_state)
  y_phase_voltage_per_switching_state8/1 -> Subsystem7/8(y_phase_voltage_per_switching_state)
  d_phase_voltage_per_switching_state9/1 -> Subsystem6/5(d_phase_voltage_per_switching_state)
  q_phase_voltage_per_switching_state9/1 -> Subsystem6/6(q_phase_voltage_per_switching_state)
  x_phase_voltage_per_switching_state9/1 -> Subsystem6/7(x_phase_voltage_per_switching_state)
  y_phase_voltage_per_switching_state9/1 -> Subsystem6/8(y_phase_voltage_per_switching_state)
  d_phase_voltage_per_switching_state10/1 -> Subsystem5/5(d_phase_voltage_per_switching_state)
  q_phase_voltage_per_switching_state10/1 -> Subsystem5/6(q_phase_voltage_per_switching_state)
  x_phase_voltage_per_switching_state10/1 -> Subsystem5/7(x_phase_voltage_per_switching_state)
  y_phase_voltage_per_switching_state10/1 -> Subsystem5/8(y_phase_voltage_per_switching_state)
  d_phase_voltage_per_switching_state11/1 -> Subsystem4/5(d_phase_voltage_per_switching_state)
  q_phase_voltage_per_switching_state11/1 -> Subsystem4/6(q_phase_voltage_per_switching_state)
  x_phase_voltage_per_switching_state11/1 -> Subsystem4/7(x_phase_voltage_per_switching_state)
  y_phase_voltage_per_switching_state11/1 -> Subsystem4/8(y_phase_voltage_per_switching_state)
  d_phase_voltage_per_switching_state12/1 -> Subsystem3/5(d_phase_voltage_per_switching_state)
  q_phase_voltage_per_switching_state12/1 -> Subsystem3/6(q_phase_voltage_per_switching_state)
  x_phase_voltage_per_switching_state12/1 -> Subsystem3/7(x_phase_voltage_per_switching_state)
  y_phase_voltage_per_switching_state12/1 -> Subsystem3/8(y_phase_voltage_per_switching_state)
  d_phase_voltage_per_switching_state13/1 -> Subsystem2/5(d_phase_voltage_per_switching_state)
  q_phase_voltage_per_switching_state13/1 -> Subsystem2/6(q_phase_voltage_per_switching_state)
  x_phase_voltage_per_switching_state13/1 -> Subsystem2/7(x_phase_voltage_per_switching_state)
  y_phase_voltage_per_switching_state13/1 -> Subsystem2/8(y_phase_voltage_per_switching_state)
  d_phase_voltage_per_switching_state14/1 -> Subsystem1/5(d_phase_voltage_per_switching_state)
  q_phase_voltage_per_switching_state14/1 -> Subsystem1/6(q_phase_voltage_per_switching_state)
  x_phase_voltage_per_switching_state14/1 -> Subsystem1/7(x_phase_voltage_per_switching_state)
  y_phase_voltage_per_switching_state14/1 -> Subsystem1/8(y_phase_voltage_per_switching_state)
  SampleTime_div_Ld15/1 -> Subsystem/1(SampleTime_div_Ld), Subsystem4/1(SampleTime_div_Ld), Subsystem7/1(SampleTime_div_Ld), Subsystem15/1(SampleTime_div_Ld), Subsystem14/1(SampleTime_div_Ld), Subsystem13/1(SampleTime_div_Ld), Subsystem12/1(SampleTime_div_Ld), Subsystem11/1(SampleTime_div_Ld), Subsystem10/1(SampleTime_div_Ld), Subsystem9/1(SampleTime_div_Ld), Subsystem8/1(SampleTime_div_Ld), Subsystem6/1(SampleTime_div_Ld), Subsystem5/1(SampleTime_div_Ld), Subsystem3/1(SampleTime_div_Ld), Subsystem2/1(SampleTime_div_Ld), Subsystem1/1(SampleTime_div_Ld)
  SampleTime_div_Lq15/1 -> Subsystem/2(SampleTime_div_Lq), Subsystem4/2(SampleTime_div_Lq), Subsystem15/2(SampleTime_div_Lq), Subsystem14/2(SampleTime_div_Lq), Subsystem13/2(SampleTime_div_Lq), Subsystem12/2(SampleTime_div_Lq), Subsystem11/2(SampleTime_div_Lq), Subsystem10/2(SampleTime_div_Lq), Subsystem9/2(SampleTime_div_Lq), Subsystem8/2(SampleTime_div_Lq), Subsystem7/2(SampleTime_div_Lq), Subsystem6/2(SampleTime_div_Lq), Subsystem5/2(SampleTime_div_Lq), Subsystem3/2(SampleTime_div_Lq), Subsystem2/2(SampleTime_div_Lq), Subsystem1/2(SampleTime_div_Lq)
  SampleTime_div_Lx15/1 -> Subsystem/3(SampleTime_div_Lx), Subsystem15/3(SampleTime_div_Lx), Subsystem14/3(SampleTime_div_Lx), Subsystem13/3(SampleTime_div_Lx), Subsystem12/3(SampleTime_div_Lx), Subsystem11/3(SampleTime_div_Lx), Subsystem10/3(SampleTime_div_Lx), Subsystem9/3(SampleTime_div_Lx), Subsystem8/3(SampleTime_div_Lx), Subsystem7/3(SampleTime_div_Lx), Subsystem6/3(SampleTime_div_Lx), Subsystem5/3(SampleTime_div_Lx), Subsystem4/3(SampleTime_div_Lx), Subsystem3/3(SampleTime_div_Lx), Subsystem2/3(SampleTime_div_Lx), Subsystem1/3(SampleTime_div_Lx)
  SampleTime_div_Ly15/1 -> Subsystem15/4(SampleTime_div_Ly), Subsystem14/4(SampleTime_div_Ly), Subsystem13/4(SampleTime_div_Ly), Subsystem12/4(SampleTime_div_Ly), Subsystem11/4(SampleTime_div_Ly), Subsystem10/4(SampleTime_div_Ly), Subsystem9/4(SampleTime_div_Ly), Subsystem8/4(SampleTime_div_Ly), Subsystem7/4(SampleTime_div_Ly), Subsystem6/4(SampleTime_div_Ly), Subsystem5/4(SampleTime_div_Ly), Subsystem4/4(SampleTime_div_Ly), Subsystem3/4(SampleTime_div_Ly), Subsystem2/4(SampleTime_div_Ly), Subsystem1/4(SampleTime_div_Ly), Subsystem/4(SampleTime_div_Ly)
  id_k_16/1 -> Subsystem/9(id_k), Subsystem15/9(id_k), Subsystem14/9(id_k), Subsystem13/9(id_k), Subsystem12/9(id_k), Subsystem11/9(id_k), Subsystem10/9(id_k), Subsystem9/9(id_k), Subsystem8/9(id_k), Subsystem7/9(id_k), Subsystem6/9(id_k), Subsystem5/9(id_k), Subsystem4/9(id_k), Subsystem3/9(id_k), Subsystem2/9(id_k), Subsystem1/9(id_k)
  iq_k_16/1 -> Subsystem/10(iq_k), Subsystem15/10(iq_k), Subsystem14/10(iq_k), Subsystem13/10(iq_k), Subsystem12/10(iq_k), Subsystem11/10(iq_k), Subsystem10/10(iq_k), Subsystem9/10(iq_k), Subsystem8/10(iq_k), Subsystem7/10(iq_k), Subsystem6/10(iq_k), Subsystem5/10(iq_k), Subsystem4/10(iq_k), Subsystem3/10(iq_k), Subsystem2/10(iq_k), Subsystem1/10(iq_k)
  ix_k_16/1 -> Subsystem/11(ix_k), Subsystem15/11(ix_k), Subsystem14/11(ix_k), Subsystem13/11(ix_k), Subsystem12/11(ix_k), Subsystem11/11(ix_k), Subsystem10/11(ix_k), Subsystem9/11(ix_k), Subsystem8/11(ix_k), Subsystem7/11(ix_k), Subsystem6/11(ix_k), Subsystem5/11(ix_k), Subsystem4/11(ix_k), Subsystem3/11(ix_k), Subsystem2/11(ix_k), Subsystem1/11(ix_k)
  iy_k_16/1 -> Subsystem/12(iy_k), Subsystem15/12(iy_k), Subsystem14/12(iy_k), Subsystem13/12(iy_k), Subsystem12/12(iy_k), Subsystem11/12(iy_k), Subsystem10/12(iy_k), Subsystem9/12(iy_k), Subsystem8/12(iy_k), Subsystem7/12(iy_k), Subsystem6/12(iy_k), Subsystem5/12(iy_k), Subsystem4/12(iy_k), Subsystem3/12(iy_k), Subsystem2/12(iy_k), Subsystem1/12(iy_k)
  Rs15/1 -> Subsystem/16(Rs), Subsystem7/16(Rs), Subsystem15/16(Rs), Subsystem14/16(Rs), Subsystem13/16(Rs), Subsystem12/16(Rs), Subsystem11/16(Rs), Subsystem10/16(Rs), Subsystem9/16(Rs), Subsystem8/16(Rs), Subsystem6/16(Rs), Subsystem5/16(Rs), Subsystem4/16(Rs), Subsystem3/16(Rs), Subsystem2/16(Rs), Subsystem1/16(Rs)
  omega_el15/1 -> Subsystem/17(omega_el), Subsystem15/17(omega_el), Subsystem14/17(omega_el), Subsystem13/17(omega_el), Subsystem12/17(omega_el), Subsystem11/17(omega_el), Subsystem10/17(omega_el), Subsystem9/17(omega_el), Subsystem8/17(omega_el), Subsystem7/17(omega_el), Subsystem6/17(omega_el), Subsystem5/17(omega_el), Subsystem4/17(omega_el), Subsystem3/17(omega_el), Subsystem2/17(omega_el), Subsystem1/17(omega_el)
  Lq15/1 -> Subsystem/14(Lq), Subsystem15/14(Lq), Subsystem14/14(Lq), Subsystem13/14(Lq), Subsystem12/14(Lq), Subsystem11/14(Lq), Subsystem10/14(Lq), Subsystem9/14(Lq), Subsystem8/14(Lq), Subsystem7/14(Lq), Subsystem6/14(Lq), Subsystem5/14(Lq), Subsystem4/14(Lq), Subsystem3/14(Lq), Subsystem2/14(Lq), Subsystem1/14(Lq)
  Ld15/1 -> Subsystem/15(Ld), Subsystem1/15(Ld), Subsystem15/15(Ld), Subsystem14/15(Ld), Subsystem13/15(Ld), Subsystem12/15(Ld), Subsystem11/15(Ld), Subsystem10/15(Ld), Subsystem9/15(Ld), Subsystem8/15(Ld), Subsystem7/15(Ld), Subsystem6/15(Ld), Subsystem5/15(Ld), Subsystem4/15(Ld), Subsystem3/15(Ld), Subsystem2/15(Ld)
  psiPM15/1 -> Subsystem/13(psiPM), Subsystem10/13(psiPM), Subsystem15/13(psiPM), Subsystem14/13(psiPM), Subsystem13/13(psiPM), Subsystem12/13(psiPM), Subsystem11/13(psiPM), Subsystem9/13(psiPM), Subsystem8/13(psiPM), Subsystem7/13(psiPM), Subsystem6/13(psiPM), Subsystem5/13(psiPM), Subsystem4/13(psiPM), Subsystem3/13(psiPM), Subsystem2/13(psiPM), Subsystem1/13(psiPM)
  d_phase_voltage_per_switching_state15/1 -> Subsystem/5(d_phase_voltage_per_switching_state)
  q_phase_voltage_per_switching_state15/1 -> Subsystem/6(q_phase_voltage_per_switching_state)
  x_phase_voltage_per_switching_state15/1 -> Subsystem/7(x_phase_voltage_per_switching_state)
  y_phase_voltage_per_switching_state15/1 -> Subsystem/8(y_phase_voltage_per_switching_state)

== system gm_test_prediction_without_delays/Prediction_and_cost_function1/Detect Rise Positive/Positive ==
  u : Inport  OutDataTypeStr=boolean  SampleTime=1e-08
  Compare : RelationalOperator  Operator=>  OutDataTypeStr=boolean  ZeroCross=off
  Constant : Constant  DisableCoverage=on  Value=0  OutDataTypeStr=Inherit: Inherit via back propagation  SampleTime=-1  PreserveConstantTs=on
  y : Outport  SampleTime=1e-08
  wires:
  Compare/1 -> y/1
  Constant/1 -> Compare/2
  u/1 -> Compare/1

== system gm_test_prediction_without_delays/Prediction_and_cost_function1/Detect Rise Positive1/Positive ==
  u : Inport  OutDataTypeStr=boolean  SampleTime=1e-08
  Compare : RelationalOperator  Operator=>  OutDataTypeStr=boolean  ZeroCross=off
  Constant : Constant  DisableCoverage=on  Value=0  OutDataTypeStr=Inherit: Inherit via back propagation  SampleTime=-1  PreserveConstantTs=on
  y : Outport  SampleTime=1e-08
  wires:
  Compare/1 -> y/1
  Constant/1 -> Compare/2
  u/1 -> Compare/1

== system gm_test_prediction_without_delays/Prediction_and_cost_function1/Detect Rise Positive2/Positive ==
  u : Inport  OutDataTypeStr=boolean  SampleTime=1e-08
  Compare : RelationalOperator  Operator=>  OutDataTypeStr=boolean  ZeroCross=off
  Constant : Constant  DisableCoverage=on  Value=0  OutDataTypeStr=Inherit: Inherit via back propagation  SampleTime=-1  PreserveConstantTs=on
  y : Outport  SampleTime=1e-08
  wires:
  Compare/1 -> y/1
  Constant/1 -> Compare/2
  u/1 -> Compare/1
